simulink model "AppMain"  (R2021a)
settings: Solver=FixedStepDiscrete  StartTime=0.0  StopTime=80  FixedStep=10e-3  RelTol=1e-3
PreLoadFcn:
  | AppMain_data
values from neighbouring files (symbols this model uses):
  CtrlConst = struct    [AppMain_data.m]
  TaskTimeBase = struct    [AppMain_data.m]
undefined symbols (not defined in the file or in its folder): Lock, Open, Short
libraries: simulink x27, lib1 x10
(part 2 of 3)

== system AppMain/MotorRestartAndFaultCnt/MotorFalutHandle/Subsystem1 ==
  IsMotorShort : Inport  OutDataTypeStr=boolean
  IsMotorOpenLoad : Inport  Port=2  OutDataTypeStr=boolean
  TargetSpeed : Inport  Port=3  OutDataTypeStr=int16
  RestartEnable : Inport  Port=4  OutDataTypeStr=boolean
  If : If  IfExpression=u1 ~= 0
  If Action Subsystem : Subsystem  TreatAsAtomicUnit=on
  If Action Subsystem1 : Subsystem  TreatAsAtomicUnit=on
  Logical Operator : Logic  Operator=OR  AllPortsSameDT=off  OutDataTypeStr=boolean
  Merge : Merge
  Speed : Outport  OutDataTypeStr=int16  VectorParamsAs1DForOutWhenUnconnected=off
  wires:
  IsMotorShort/1 -> Logical Operator/1
  IsMotorOpenLoad/1 -> Logical Operator/2
  Logical Operator/1 -> If/1
  TargetSpeed/1 -> If Action Subsystem1/1(SpeedIn), If Action Subsystem/1(SpeedIn)
  RestartEnable/1 -> If Action Subsystem1/2(RestartEnable)
  If/1 -> If Action Subsystem/Action
  If/2 -> If Action Subsystem1/Action
  If Action Subsystem1/1(SpeedOut) -> Merge/2
  If Action Subsystem/1(SpeedOut) -> Merge/1
  Merge/1 -> Speed/1

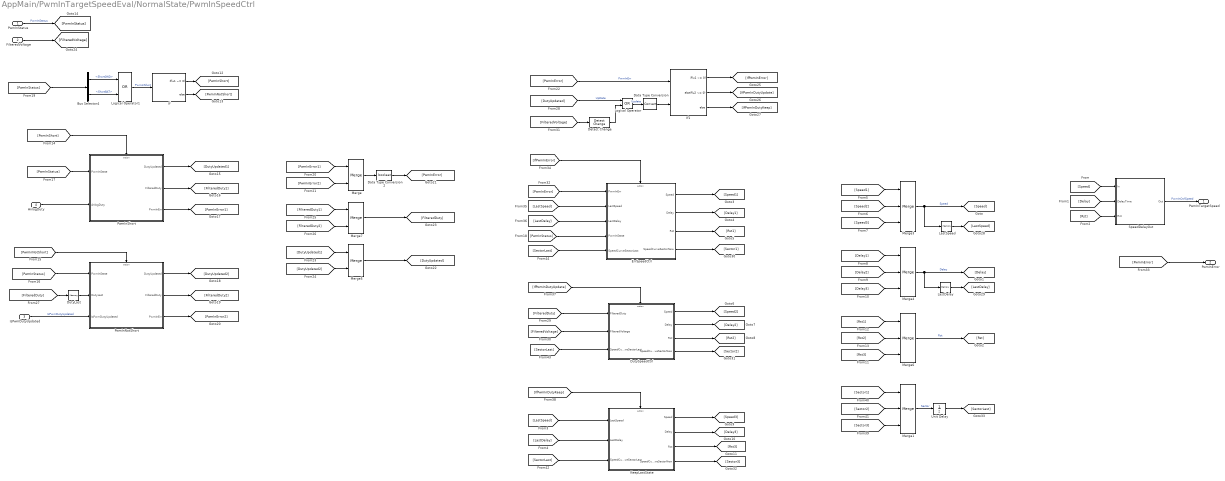
== system AppMain/PwmInTargetSpeedEval/NormalState/PwmInSpeedCtrl ==
  PwmInStatus : Inport
  FilteredVoltage : Inport  Port=2  OutDataTypeStr=int16
  IsPwmDutyUpdated : Inport  Port=3  OutDataTypeStr=boolean
  AnlogDuty : Inport  Port=4  OutDataTypeStr=uint16
  Bus Selector4 : BusSelector  OutputSignals=ShortGND,ShortBAT
  Data Type Conversion : DataTypeConversion
  Data Type Conversion2 : DataTypeConversion  OutDataTypeStr=boolean
  Detect Change : simulink/Logic and Bit Operations/Detect Change  vinit=0  OutDataTypeStr=boolean
  DutyLast : Memory  InitialCondition=CtrlConst.SpeedCtrl.PwmIn.Duty.Default  InheritSampleTime=on
  DutySpeedCtrl : Subsystem  TreatAsAtomicUnit=on
  ErrSpeedCtrl : Subsystem  TreatAsAtomicUnit=on
  If : If  IfExpression=u1 ~= 0
  If1 : If  NumInputs=2  IfExpression=u1 ~= 0  ElseIfExpressions=u2 ~= 0
  KeepLastState : Subsystem  TreatAsAtomicUnit=on
  LastDelay : Memory  InheritSampleTime=on
  LastSpeed : Memory  InheritSampleTime=on
  Logical Operator : Logic  Operator=OR  AllPortsSameDT=off  OutDataTypeStr=boolean
  Logical Operator1 : Logic  Operator=OR  AllPortsSameDT=off  OutDataTypeStr=boolean
  Merge : Merge
  Merge{1,3..4,6} (4 alike) : Merge  Inputs=3
  Merge5 : Merge
  Merge7 : Merge
  PwmInNotShort : Subsystem  TreatAsAtomicUnit=on
      settings: RTWSystemCode=Nonreusable function  RTWFcnNameOpts=Use subsystem name  FunctionInterfaceSpec=Allow arguments (Optimized)
  PwmInShort : Subsystem  TreatAsAtomicUnit=on
      settings: RTWSystemCode=Nonreusable function  RTWFcnNameOpts=Use subsystem name  FunctionInterfaceSpec=Allow arguments (Optimized)
  SpeedDelayOut : Subsystem  TreatAsAtomicUnit=on
      settings: RTWFcnNameOpts=Use subsystem name
  Unit Delay : UnitDelay  InitialCondition=CtrlConst.SpeedCtrl.DefaultSector  SampleTime=-1  HasFrameUpgradeWarning=on
  PwmInTargetSpeed : Outport  VectorParamsAs1DForOutWhenUnconnected=off
  PwmInError : Outport  Port=2  OutDataTypeStr=boolean  VectorParamsAs1DForOutWhenUnconnected=off
  wires:
  SpeedDelayOut/1(Out) -> PwmInTargetSpeed/1  "PwmInCtrlSpeed"
  PwmInStatus/1 -> [PwmInStatus]  "PwmInStatus"
  Bus Selector4/1 -> Logical Operator1/1  "<ShortGND>"
  Bus Selector4/2 -> Logical Operator1/2  "<ShortBAT>"
  Logical Operator1/1 -> If/1  "PwmInShort"
  [PwmInShort] -> PwmInShort/Action
  [PwmInNotShort] -> PwmInNotShort/Action
  [FilteredDuty] -> DutySpeedCtrl/1(FilteredDuty)
  Merge3/1 -> LastSpeed/1, [Speed]  "Speed"
  Merge4/1 -> LastDelay/1, [Delay]  "Delay"
  [DutyUpdated] -> Logical Operator/1  "UpDate"
  [LastDelay] -> KeepLastState/2(LastDelay)
  [LastSpeed] -> KeepLastState/1(LastSpeed)
  [PwmInError] -> If1/1  "PwmInErr"
  Data Type Conversion/1 -> If1/2
  DutyLast/1 -> PwmInNotShort/2(DutyLast)
  [FilteredVoltage] -> DutySpeedCtrl/2(FilteredVoltage)
  Merge/1 -> Data Type Conversion2/1
  Logical Operator/1 -> Data Type Conversion/1  "Update"
  IsPwmDutyUpdated/1 -> PwmInNotShort/3(IsPwmDutyUpdated)  "IsPwmDutyUpdated"
  AnlogDuty/1 -> PwmInShort/2(AnlogDuty)
  Merge6/1 -> [Rst]  "Rst"
  [Speed] -> SpeedDelayOut/1(In)
  [Delay] -> SpeedDelayOut/2(DelayTime)
  [Rst] -> SpeedDelayOut/3(Rst)
  ErrSpeedCtrl/1(Speed) -> [Speed1]
  ErrSpeedCtrl/2(Delay) -> [Delay1]
  ErrSpeedCtrl/3(Rst) -> [Rst1]
  DutySpeedCtrl/1(Speed) -> [Speed2]
  DutySpeedCtrl/2(Delay) -> [Delay2]
  DutySpeedCtrl/3(Rst) -> [Rst2]
  KeepLastState/1(Speed) -> [Speed3]
  KeepLastState/2(Delay) -> [Delay3]
  KeepLastState/3(Rst) -> [Rst3]
  [Speed1] -> Merge3/1
  [Speed2] -> Merge3/2
  [Speed3] -> Merge3/3
  [Delay1] -> Merge4/1
  [Delay2] -> Merge4/2
  [Delay3] -> Merge4/3
  [Rst3] -> Merge6/3
  [Rst2] -> Merge6/2
  [Rst1] -> Merge6/1
  If/1 -> [PwmInShort]
  If/2 -> [PwmInNotShort]
  [PwmInStatus] -> PwmInNotShort/1(PwmInState)
  [PwmInStatus] -> ErrSpeedCtrl/4(PwmInState)
  [PwmInStatus] -> PwmInShort/1(PwmInState)
  [PwmInStatus] -> Bus Selector4/1
  PwmInShort/3(PwmInErr) -> [PwmInError1]
  PwmInShort/2(FilteredDuty) -> [FilteredDuty1]
  PwmInShort/1(DutyUpdated) -> [DutyUpdated1]
  PwmInNotShort/1(DutyUpdated) -> [DutyUpdated2]
  PwmInNotShort/2(FilteredDuty) -> [FilteredDuty2]
  PwmInNotShort/3(PwmInErr) -> [PwmInError2]
  [PwmInError1] -> Merge/1
  [PwmInError2] -> Merge/2
  [DutyUpdated2] -> Merge5/2
  [DutyUpdated1] -> Merge5/1
  Merge5/1 -> [DutyUpdated]
  Merge7/1 -> [FilteredDuty]
  [FilteredDuty1] -> Merge7/1
  [FilteredDuty2] -> Merge7/2
  [FilteredDuty] -> DutyLast/1
  [FilteredVoltage] -> Detect Change/1
  Detect Change/1 -> Logical Operator/2
  FilteredVoltage/1 -> [FilteredVoltage]
  Data Type Conversion2/1 -> [PwmInError]
  [PwmInError] -> ErrSpeedCtrl/1(PwmInErr)
  [PwmInError] -> PwmInError/1
  If1/1 -> [IfPwmInError]
  If1/2 -> [IfPwmInDutyUpdate]
  If1/3 -> [IfPwmInDutyKeep]
  [IfPwmInError] -> ErrSpeedCtrl/Action
  LastSpeed/1 -> [LastSpeed]
  LastDelay/1 -> [LastDelay]
  [LastSpeed] -> ErrSpeedCtrl/2(LastSpeed)
  [LastDelay] -> ErrSpeedCtrl/3(LastDelay)
  ErrSpeedCtrl/4(SpeedCurveSectorNew) -> [Sector1]
  [IfPwmInDutyUpdate] -> DutySpeedCtrl/Action
  DutySpeedCtrl/4(SpeedCurveSectorNew) -> [Sector2]
  [IfPwmInDutyKeep] -> KeepLastState/Action
  KeepLastState/4(SpeedCurveSectorNew) -> [Sector3]
  [Sector1] -> Merge1/1
  [Sector2] -> Merge1/2
  [Sector3] -> Merge1/3
  Merge1/1 -> Unit Delay/1  "Sector"
  Unit Delay/1 -> [SectorLast]
  [SectorLast] -> KeepLastState/3(SpeedCurveSectorLast)
  [SectorLast] -> DutySpeedCtrl/3(SpeedCurveSectorLast)
  [SectorLast] -> ErrSpeedCtrl/5(SpeedCurveSectorLast)

== system AppMain/FeedBack/Subsystem7/Subsystem10/Subsystem1 ==
  Status : Inport
  Compare To Zero : simulink/Logic and Bit Operations/Compare To Zero  relop=~=  OutDataTypeStr=boolean
  Constant1 : Constant  Value=CtrlConst.FeedBack.EndDelay.Voltage  OutDataTypeStr=uint16
  Constant2 : Constant  Value=CtrlConst.FeedBack.StartDelay.Voltage  OutDataTypeStr=uint16
  Display : Display
  Display1 : Display
  FeedBackDelay4 : lib1/FeedBackDelay  SystemSampleTime=-1  VariantActivationTime=update diagram  Latency=0  AutoFrameSizeCalculation=off
      settings: SourceProductName=lib1
  FeedBackFlag : Outport  VectorParamsAs1DForOutWhenUnconnected=off
  wires:
  FeedBackDelay4/1 -> FeedBackFlag/1  "FeedBackFlag"
  Constant1/1 -> Display1/1, FeedBackDelay4/3
  Constant2/1 -> Display/1, FeedBackDelay4/1
  Compare To Zero/1 -> FeedBackDelay4/2
  Status/1 -> Compare To Zero/1

== system AppMain/FeedBack/Subsystem7/Subsystem10/Subsystem2 ==
  Status : Inport
  Compare To Zero : simulink/Logic and Bit Operations/Compare To Zero  relop=>  OutDataTypeStr=boolean
  Constant1 : Constant  Value=CtrlConst.FeedBack.EndDelay.AmbT  OutDataTypeStr=uint16
  Constant2 : Constant  Value=CtrlConst.FeedBack.StartDelay.AmbT  OutDataTypeStr=uint16
  Display : Display
  Display1 : Display
  FeedBackDelay4 : lib1/FeedBackDelay  SystemSampleTime=-1  VariantActivationTime=update diagram  Latency=0  AutoFrameSizeCalculation=off
      settings: SourceProductName=lib1
  FeedBackFlag : Outport  VectorParamsAs1DForOutWhenUnconnected=off
  wires:
  Status/1 -> Compare To Zero/1
  Compare To Zero/1 -> FeedBackDelay4/2
  Constant2/1 -> FeedBackDelay4/1, Display/1
  Constant1/1 -> FeedBackDelay4/3, Display1/1
  FeedBackDelay4/1 -> FeedBackFlag/1  "FeedBackFlag"

== system AppMain/FeedBack/Subsystem7/Subsystem10/Subsystem6 ==
  Status : Inport
  Compare To Zero : simulink/Logic and Bit Operations/Compare To Zero  relop=~=  OutDataTypeStr=boolean
  Constant1 : Constant  Value=CtrlConst.FeedBack.EndDelay.AmbTPreOver  OutDataTypeStr=uint16
  Constant2 : Constant  Value=CtrlConst.FeedBack.StartDelay.AmbTPreOver  OutDataTypeStr=uint16
  Display : Display
  Display1 : Display
  FeedBackDelay4 : lib1/FeedBackDelay  SystemSampleTime=-1  VariantActivationTime=update diagram  Latency=0  AutoFrameSizeCalculation=off
      settings: SourceProductName=lib1
  FeedBackFlag : Outport  VectorParamsAs1DForOutWhenUnconnected=off
  wires:
  Status/1 -> Compare To Zero/1
  Compare To Zero/1 -> FeedBackDelay4/2
  Constant2/1 -> FeedBackDelay4/1, Display/1
  Constant1/1 -> FeedBackDelay4/3, Display1/1
  FeedBackDelay4/1 -> FeedBackFlag/1  "FeedBackFlag"

== system AppMain/FeedBack/Subsystem7/Subsystem10/Subsystem7 ==
  Status : Inport
  Compare To Zero : simulink/Logic and Bit Operations/Compare To Zero  relop=~=  OutDataTypeStr=boolean
  Constant1 : Constant  Value=CtrlConst.FeedBack.EndDelay.MotorShort  OutDataTypeStr=uint16
  Constant2 : Constant  Value=CtrlConst.FeedBack.StartDelay.MotorShort  OutDataTypeStr=uint16
  Display : Display
  Display1 : Display
  FeedBackDelay4 : lib1/FeedBackDelay  SystemSampleTime=-1  VariantActivationTime=update diagram  Latency=0  AutoFrameSizeCalculation=off
      settings: SourceProductName=lib1
  FeedBackFlag : Outport  VectorParamsAs1DForOutWhenUnconnected=off
  wires:
  FeedBackDelay4/1 -> FeedBackFlag/1  "FeedBackFlag"
  Constant1/1 -> Display1/1, FeedBackDelay4/3
  Constant2/1 -> Display/1, FeedBackDelay4/1
  Compare To Zero/1 -> FeedBackDelay4/2
  Status/1 -> Compare To Zero/1

== system AppMain/FeedBack/Subsystem7/Subsystem10/Subsystem8 ==
  Status : Inport
  Compare To Zero : simulink/Logic and Bit Operations/Compare To Zero  relop=~=  OutDataTypeStr=boolean
  Constant1 : Constant  Value=CtrlConst.FeedBack.EndDelay.MotorOpenLoad  OutDataTypeStr=uint16
  Constant2 : Constant  Value=CtrlConst.FeedBack.StartDelay.MotorOpenLoad  OutDataTypeStr=uint16
  Display : Display
  Display1 : Display
  FeedBackDelay4 : lib1/FeedBackDelay  SystemSampleTime=-1  VariantActivationTime=update diagram  Latency=0  AutoFrameSizeCalculation=off
      settings: SourceProductName=lib1
  FeedBackFlag : Outport  VectorParamsAs1DForOutWhenUnconnected=off
  wires:
  Status/1 -> Compare To Zero/1
  Compare To Zero/1 -> FeedBackDelay4/2
  Constant2/1 -> FeedBackDelay4/1, Display/1
  Constant1/1 -> FeedBackDelay4/3, Display1/1
  FeedBackDelay4/1 -> FeedBackFlag/1  "FeedBackFlag"

== system AppMain/FeedBack/Subsystem7/Subsystem10/Subsystem9 ==
  Status : Inport
  Compare To Zero : simulink/Logic and Bit Operations/Compare To Zero  relop=~=  OutDataTypeStr=boolean
  Constant1 : Constant  Value=CtrlConst.FeedBack.EndDelay.MotorLock  OutDataTypeStr=uint16
  Constant2 : Constant  Value=CtrlConst.FeedBack.StartDelay.MotorLock  OutDataTypeStr=uint16
  Display : Display
  Display1 : Display
  FeedBackDelay4 : lib1/FeedBackDelay  SystemSampleTime=-1  VariantActivationTime=update diagram  Latency=0  AutoFrameSizeCalculation=off
      settings: SourceProductName=lib1
  FeedBackFlag : Outport  VectorParamsAs1DForOutWhenUnconnected=off
  wires:
  FeedBackDelay4/1 -> FeedBackFlag/1  "FeedBackFlag"
  Constant1/1 -> Display1/1, FeedBackDelay4/3
  Constant2/1 -> Display/1, FeedBackDelay4/1
  Compare To Zero/1 -> FeedBackDelay4/2
  Status/1 -> Compare To Zero/1

== system AppMain/MotorRestartAndFaultCnt/MotorFalutHandle/Subsystem/If Action Subsystem ==
  FalutCntLast : Inport  OutDataTypeStr=Bus: MotorFaultCnt_t
  IsMotorShort : Inport  Port=2  OutDataTypeStr=boolean
  IsMotorLock : Inport  Port=3  OutDataTypeStr=boolean
  IsMotorOpenLoad : Inport  Port=4  OutDataTypeStr=boolean
  Action Port : ActionPort  InitializeStates=reset  ActionPortLabel=if(u1 ~= 0)
  FaultCntIncrement : Subsystem
  RestartIntervalCaculate : Subsystem
  FaultCnt : Outport  OutDataTypeStr=Bus: MotorFaultCnt_t  VectorParamsAs1DForOutWhenUnconnected=off
  RestartInterval : Outport  Port=2  OutDataTypeStr=uint16  VectorParamsAs1DForOutWhenUnconnected=off
  wires:
  FaultCntIncrement/1(FaultCnt) -> RestartIntervalCaculate/1(MotorFaultCnt), FaultCnt/1
  FalutCntLast/1 -> FaultCntIncrement/1(FalutCntLast)
  IsMotorShort/1 -> FaultCntIncrement/2(IsMotorShort)
  RestartIntervalCaculate/1(TimeTHR) -> RestartInterval/1
  IsMotorOpenLoad/1 -> FaultCntIncrement/3(IsMotorOpenLoad)
  IsMotorLock/1 -> FaultCntIncrement/4(IsMotorLock)

== system AppMain/MotorRestartAndFaultCnt/MotorFalutHandle/Subsystem/If Action Subsystem1 ==
  FaultCntLast : Inport  OutDataTypeStr=Bus: MotorFaultCnt_t
  RestartIntervalLast : Inport  Port=2  OutDataTypeStr=uint16
  Action Port : ActionPort  InitializeStates=reset  ActionPortLabel=else
  Bus Creator : BusCreator  Inputs=3  OutDataTypeStr=Bus: MotorFaultCnt_t  NonVirtualBus=on
      settings: InheritFromInputs=off
  Bus Selector : BusSelector  OutputSignals=Short,Open,Lock
  FaultCnt : Outport  OutDataTypeStr=Bus: MotorFaultCnt_t  VectorParamsAs1DForOutWhenUnconnected=off
  RestartInterval : Outport  Port=2  OutDataTypeStr=uint16  VectorParamsAs1DForOutWhenUnconnected=off
  wires:
  FaultCntLast/1 -> Bus Selector/1
  Bus Creator/1 -> FaultCnt/1
  Bus Selector/1 -> Bus Creator/1  "<Short>"
  Bus Selector/2 -> Bus Creator/2  "<Open>"
  Bus Selector/3 -> Bus Creator/3  "<Lock>"
  RestartIntervalLast/1 -> RestartInterval/1

== system AppMain/MotorRestartAndFaultCnt/MotorFalutHandle/Subsystem1/If Action Subsystem ==
  SpeedIn : Inport
  Action Port : ActionPort  ActionPortLabel=if(u1 ~= 0)
  SpeedOut : Outport  VectorParamsAs1DForOutWhenUnconnected=off
  wires:
  SpeedIn/1 -> SpeedOut/1

== system AppMain/MotorRestartAndFaultCnt/MotorFalutHandle/Subsystem1/If Action Subsystem1 ==
  SpeedIn : Inport
  RestartEnable : Inport  Port=2  OutDataTypeStr=boolean
  Action Port : ActionPort  InitializeStates=reset  ActionPortLabel=else
  Terminator : Terminator
  SpeedOut : Outport  VectorParamsAs1DForOutWhenUnconnected=off
  wires:
  SpeedIn/1 -> SpeedOut/1
  RestartEnable/1 -> Terminator/1

== system AppMain/PwmInTargetSpeedEval/NormalState/PwmInSpeedCtrl/DutySpeedCtrl ==
  FilteredDuty : Inport  OutDataTypeStr=uint16
  FilteredVoltage : Inport  Port=2  OutDataTypeStr=int16
  SpeedCurveSectorLast : Inport  Port=3
  Action Port : ActionPort  InitializeStates=reset  ActionPortLabel=elseif(u2 ~= 0)
  SpeedAndOutDelayEval : Subsystem
      settings: RTWFcnNameOpts=Use subsystem name
  Speed : Outport  OutDataTypeStr=int16  VectorParamsAs1DForOutWhenUnconnected=off
  Delay : Outport  Port=2  OutDataTypeStr=uint16  VectorParamsAs1DForOutWhenUnconnected=off
  Rst : Outport  Port=3  OutDataTypeStr=boolean  VectorParamsAs1DForOutWhenUnconnected=off
  SpeedCurveSectorNew : Outport  Port=4
  wires:
  FilteredDuty/1 -> SpeedAndOutDelayEval/1(FilteredDuty)
  SpeedAndOutDelayEval/1(DutySpeed) -> Speed/1  "Speed"
  SpeedAndOutDelayEval/2(DelayTime) -> Delay/1  "Delay"
  SpeedAndOutDelayEval/3(DelayRst) -> Rst/1  "Rst"
  FilteredVoltage/1 -> SpeedAndOutDelayEval/2(FilteredVoltage)
  SpeedCurveSectorLast/1 -> SpeedAndOutDelayEval/3(SpeedCurveSectorLast)
  SpeedAndOutDelayEval/4(SpeedCurveSectorNew) -> SpeedCurveSectorNew/1

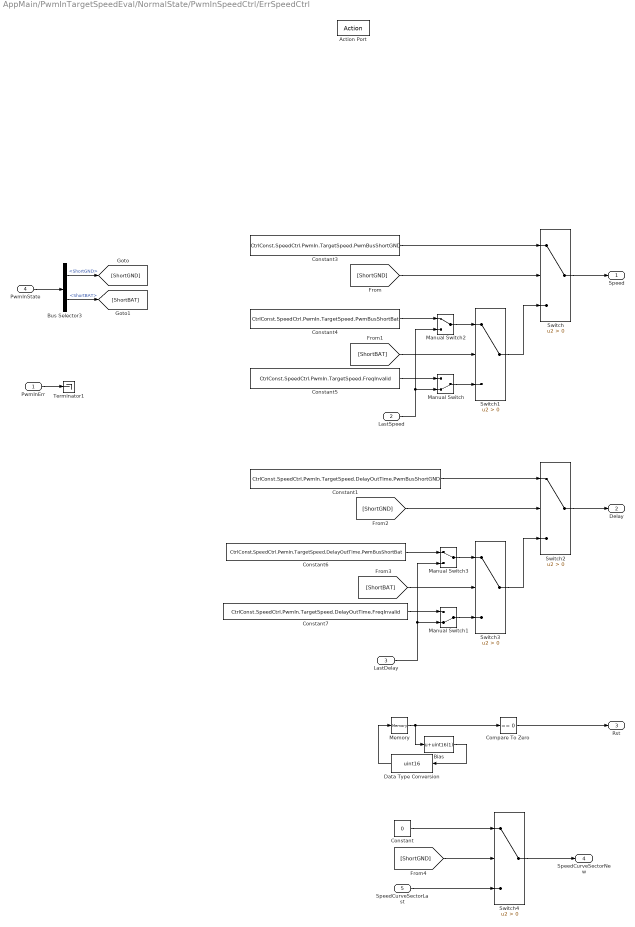
== system AppMain/PwmInTargetSpeedEval/NormalState/PwmInSpeedCtrl/ErrSpeedCtrl ==
  PwmInErr : Inport  OutDataTypeStr=boolean
  LastSpeed : Inport  Port=2  OutDataTypeStr=int16
  LastDelay : Inport  Port=3  OutDataTypeStr=uint16
  PwmInState : Inport  Port=4
  SpeedCurveSectorLast : Inport  Port=5
  Action Port : ActionPort  InitializeStates=reset  ActionPortLabel=if(u1 ~= 0)
  Bias : Bias  Bias=uint16(1)
  Bus Selector3 : BusSelector  OutputSignals=ShortGND,ShortBAT
  Compare To Zero : simulink/Logic and Bit Operations/Compare To Zero  relop===  OutDataTypeStr=boolean
  Constant : Constant  Value=0  OutDataTypeStr=uint16
  Constant1 : Constant  Value=CtrlConst.SpeedCtrl.PwmIn.TargetSpeed.DelayOutTime.PwmBusShortGND
  Constant3 : Constant  Value=CtrlConst.SpeedCtrl.PwmIn.TargetSpeed.PwmBusShortGND
  Constant4 : Constant  Value=CtrlConst.SpeedCtrl.PwmIn.TargetSpeed.PwmBusShortBat
  Constant5 : Constant  Value=CtrlConst.SpeedCtrl.PwmIn.TargetSpeed.FreqInvalid
  Constant6 : Constant  Value=CtrlConst.SpeedCtrl.PwmIn.TargetSpeed.DelayOutTime.PwmBusShortBat
  Constant7 : Constant  Value=CtrlConst.SpeedCtrl.PwmIn.TargetSpeed.DelayOutTime.FreqInvalid
  Data Type Conversion : DataTypeConversion  OutDataTypeStr=uint16
  Manual Switch : ManualSwitch  CurrentSetting=0
  Manual Switch1 : ManualSwitch  CurrentSetting=0
  Manual Switch2 : ManualSwitch
  Manual Switch3 : ManualSwitch
  Memory : Memory  InitialCondition=uint16(0)  InheritSampleTime=on
  Switch{,1..4} (5 alike) : Switch  Criteria=u2 > Threshold
  Terminator1 : Terminator
  Speed : Outport  OutDataTypeStr=int16  VectorParamsAs1DForOutWhenUnconnected=off
  Delay : Outport  Port=2  OutDataTypeStr=uint16  VectorParamsAs1DForOutWhenUnconnected=off
  Rst : Outport  Port=3  OutDataTypeStr=boolean  VectorParamsAs1DForOutWhenUnconnected=off
  SpeedCurveSectorNew : Outport  Port=4  OutDataTypeStr=uint16
  wires:
  PwmInState/1 -> Bus Selector3/1
  Constant3/1 -> Switch/1
  Switch1/1 -> Switch/3
  Switch/1 -> Speed/1
  Switch3/1 -> Switch2/3
  Constant1/1 -> Switch2/1
  Switch2/1 -> Delay/1
  Data Type Conversion/1 -> Memory/1
  Bias/1 -> Data Type Conversion/1
  Memory/1 -> Bias/1, Compare To Zero/1
  Compare To Zero/1 -> Rst/1
  LastSpeed/1 -> Manual Switch2/2, Manual Switch/2
  LastDelay/1 -> Manual Switch3/2, Manual Switch1/2
  Constant4/1 -> Manual Switch2/1
  PwmInErr/1 -> Terminator1/1
  Manual Switch/1 -> Switch1/3
  Constant5/1 -> Manual Switch/1
  Constant7/1 -> Manual Switch1/1
  Manual Switch1/1 -> Switch3/3
  Manual Switch2/1 -> Switch1/1
  Constant6/1 -> Manual Switch3/1
  Switch4/1 -> SpeedCurveSectorNew/1
  Bus Selector3/1 -> [ShortGND]  "<ShortGND>"
  Bus Selector3/2 -> [ShortBAT]  "<ShortBAT>"
  [ShortGND] -> Switch/2
  [ShortBAT] -> Switch1/2
  [ShortGND] -> Switch2/2
  [ShortBAT] -> Switch3/2
  [ShortGND] -> Switch4/2
  Constant/1 -> Switch4/1
  SpeedCurveSectorLast/1 -> Switch4/3
  Manual Switch3/1 -> Switch3/1

== system AppMain/PwmInTargetSpeedEval/NormalState/PwmInSpeedCtrl/KeepLastState ==
  LastSpeed : Inport  OutDataTypeStr=int16
  LastDelay : Inport  Port=2  OutDataTypeStr=uint16
  SpeedCurveSectorLast : Inport  Port=3  OutDataTypeStr=uint16
  Action Port : ActionPort  InitializeStates=reset  ActionPortLabel=else
  Constant : Constant  Value=false  OutDataTypeStr=boolean
  Speed : Outport  OutDataTypeStr=int16  VectorParamsAs1DForOutWhenUnconnected=off
  Delay : Outport  Port=2  OutDataTypeStr=uint16  VectorParamsAs1DForOutWhenUnconnected=off
  Rst : Outport  Port=3  OutDataTypeStr=boolean  VectorParamsAs1DForOutWhenUnconnected=off
  SpeedCurveSectorNew : Outport  Port=4  OutDataTypeStr=uint16
  wires:
  LastSpeed/1 -> Speed/1
  LastDelay/1 -> Delay/1
  Constant/1 -> Rst/1
  SpeedCurveSectorLast/1 -> SpeedCurveSectorNew/1

== system AppMain/PwmInTargetSpeedEval/NormalState/PwmInSpeedCtrl/PwmInNotShort ==
  PwmInState : Inport
  DutyLast : Inport  Port=2  OutDataTypeStr=uint16
  IsPwmDutyUpdated : Inport  Port=3  OutDataTypeStr=boolean
  Action Port : ActionPort  InitializeStates=reset  ActionPortLabel=else
  Bus Selector2 : BusSelector  OutputSignals=Freq,HighDuty
  Detect Increase : simulink/Logic and Bit Operations/Detect Increase  vinit=0.0  OutDataTypeStr=boolean
  DutyFilter : Subsystem  TreatAsAtomicUnit=on
      settings: RTWFcnNameOpts=Use subsystem name
  FreqValidJudge : Subsystem  TreatAsAtomicUnit=on
      settings: RTWFcnNameOpts=Use subsystem name
  Logical Operator : Logic  Operator=OR  AllPortsSameDT=off  OutDataTypeStr=boolean
  Logical Operator2 : Logic  Operator=NOT  Inputs=3  AllPortsSameDT=off  OutDataTypeStr=boolean
  Relational Operator : RelationalOperator  Operator=~=  OutDataTypeStr=boolean  RndMeth=Simplest
  Switch : Switch  Criteria=u2 > Threshold
  DutyUpdated : Outport  OutDataTypeStr=boolean  VectorParamsAs1DForOutWhenUnconnected=off
  FilteredDuty : Outport  Port=2  OutDataTypeStr=uint16  VectorParamsAs1DForOutWhenUnconnected=off
  PwmInErr : Outport  Port=3  OutDataTypeStr=boolean  VectorParamsAs1DForOutWhenUnconnected=off
  wires:
  Detect Increase/1 -> Logical Operator/1
  DutyFilter/2(Valid) -> Detect Increase/1  "Valid"
  PwmInState/1 -> Bus Selector2/1
  Bus Selector2/2 -> DutyFilter/1(Duty)  "<HighDuty>"
  Bus Selector2/1 -> FreqValidJudge/1(Freq)  "<Freq>"
  DutyFilter/1(FilteredDuty) -> Relational Operator/1, Switch/1  "FilteredDuty"
  Logical Operator2/1 -> PwmInErr/1  "FreqInvalid"
  FreqValidJudge/1(Valid) -> Logical Operator2/1, Switch/2, DutyFilter/Enable  "FreqValid"
  Relational Operator/1 -> Logical Operator/2
  Logical Operator/1 -> DutyUpdated/1  "UpdateFlag"
  IsPwmDutyUpdated/1 -> DutyFilter/3(IsPwmDutyUpdated)  "IsPwmDutyUpdated"
  Switch/1 -> FilteredDuty/1
  DutyLast/1 -> Relational Operator/2, Switch/3, DutyFilter/2(DutyLast)  "FilteredDuty"

== system AppMain/PwmInTargetSpeedEval/NormalState/PwmInSpeedCtrl/PwmInShort ==
  PwmInState : Inport
  AnlogDuty : Inport  Port=2  OutDataTypeStr=uint16
  Action Port : ActionPort  InitializeStates=reset  ActionPortLabel=if(u1 ~= 0)
  Bus Selector3 : BusSelector  OutputSignals=ShortGND,ShortBAT
  Constant : Constant  Value=true  OutDataTypeStr=boolean
  Detect Change : simulink/Logic and Bit Operations/Detect Change  vinit=0  OutDataTypeStr=boolean
  Detect Increase : simulink/Logic and Bit Operations/Detect Increase  vinit=0.0  OutDataTypeStr=boolean
  Detect Increase1 : simulink/Logic and Bit Operations/Detect Increase  vinit=0.0  OutDataTypeStr=boolean
  Duty0 : Constant  Value=0  OutDataTypeStr=uint16
  Duty100 : Constant  Value=1000  OutDataTypeStr=uint16
  Logical Operator3 : Logic  Operator=OR  Inputs=3  AllPortsSameDT=off  OutDataTypeStr=boolean
  Manual Switch : ManualSwitch  CurrentSetting=0
  Switch : Switch  Criteria=u2 > Threshold
  DutyUpdated : Outport  OutDataTypeStr=boolean  VectorParamsAs1DForOutWhenUnconnected=off
  FilteredDuty : Outport  Port=2  OutDataTypeStr=uint16  VectorParamsAs1DForOutWhenUnconnected=off
  PwmInErr : Outport  Port=3  OutDataTypeStr=boolean  VectorParamsAs1DForOutWhenUnconnected=off
  wires:
  Switch/1 -> FilteredDuty/1  "FilteredDuty"
  Logical Operator3/1 -> DutyUpdated/1  "DutyUpdate"
  Bus Selector3/2 -> Detect Increase1/1, Switch/2  "<ShortBAT>"
  Bus Selector3/1 -> Detect Increase/1  "<ShortGND>"
  Detect Increase1/1 -> Logical Operator3/2
  Detect Increase/1 -> Logical Operator3/1
  Duty0/1 -> Switch/1
  PwmInState/1 -> Bus Selector3/1
  Constant/1 -> PwmInErr/1
  AnlogDuty/1 -> Manual Switch/1, Detect Change/1
  Detect Change/1 -> Logical Operator3/3
  Manual Switch/1 -> Switch/3
  Duty100/1 -> Manual Switch/2

== system AppMain/PwmInTargetSpeedEval/NormalState/PwmInSpeedCtrl/SpeedDelayOut ==
  In : Inport
  DelayTime : Inport  Port=2
  Rst : Inport  Port=3
  DelayOut : Stateflow chart  TreatAsAtomicUnit=on
  OutLast : Memory  InheritSampleTime=on
  Out : Outport  VectorParamsAs1DForOutWhenUnconnected=off
  wires:
  In/1 -> DelayOut/1(In)  "In"
  OutLast/1 -> DelayOut/4(OutLast)  "OutLast"
  Rst/1 -> DelayOut/3(Rst)  "Rst"
  DelayOut/1(Out) -> OutLast/1, Out/1  "Out"
  DelayTime/1 -> DelayOut/2(DelayTHR)  "DelayTHR"

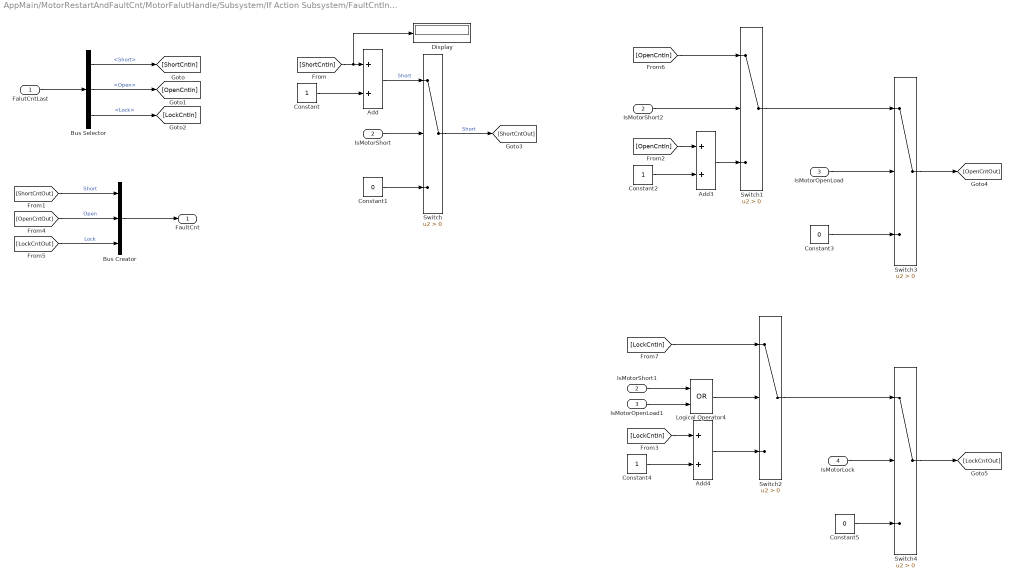
== system AppMain/MotorRestartAndFaultCnt/MotorFalutHandle/Subsystem/If Action Subsystem/FaultCntIncrement ==
  FalutCntLast : Inport  OutDataTypeStr=Bus: MotorFaultCnt_t
  IsMotorShort : Inport  Port=2  OutDataTypeStr=boolean
  IsMotorOpenLoad : Inport  Port=3  OutDataTypeStr=boolean
  IsMotorLock : Inport  Port=4  OutDataTypeStr=boolean
  Add : Sum  SaturateOnIntegerOverflow=on
  Add3 : Sum  SaturateOnIntegerOverflow=on
  Add4 : Sum  SaturateOnIntegerOverflow=on
  Bus Creator : BusCreator  Inputs=Short,Open,Lock  OutDataTypeStr=Bus: MotorFaultCnt_t  NonVirtualBus=on
  Bus Selector : BusSelector  OutputSignals=Short,Open,Lock
  Constant : Constant  OutDataTypeStr=uint8
  Constant1 : Constant  Value=0  OutDataTypeStr=uint8
  Constant2 : Constant  OutDataTypeStr=uint8
  Constant3 : Constant  Value=0  OutDataTypeStr=uint8
  Constant4 : Constant  OutDataTypeStr=uint8
  Constant5 : Constant  Value=0  OutDataTypeStr=uint8
  Display : Display
  IsMotorOpenLoad1 : InportShadow  Port=3  OutDataTypeStr=boolean
  IsMotorShort1 : InportShadow  Port=2  OutDataTypeStr=boolean
  IsMotorShort2 : InportShadow  Port=2  OutDataTypeStr=boolean
  Logical Operator4 : Logic  Operator=OR  AllPortsSameDT=off  OutDataTypeStr=boolean
  Switch{,1..4} (5 alike) : Switch  Criteria=u2 > Threshold
  FaultCnt : Outport  OutDataTypeStr=Bus: MotorFaultCnt_t  VectorParamsAs1DForOutWhenUnconnected=off
  wires:
  Bus Creator/1 -> FaultCnt/1
  Constant/1 -> Add/2
  Bus Selector/2 -> [OpenCntIn]  "<Open>"
  Bus Selector/1 -> [ShortCntIn]  "<Short>"
  Constant1/1 -> Switch/3
  Add/1 -> Switch/1  "Short"
  FalutCntLast/1 -> Bus Selector/1
  IsMotorShort/1 -> Switch/2
  Bus Selector/3 -> [LockCntIn]  "<Lock>"
  [ShortCntIn] -> Display/1, Add/1
  Switch/1 -> [ShortCntOut]  "Short"
  [ShortCntOut] -> Bus Creator/1  "Short"
  Add3/1 -> Switch1/3
  Constant2/1 -> Add3/2
  [OpenCntIn] -> Add3/1
  Constant3/1 -> Switch3/3
  Switch3/1 -> [OpenCntOut]
  IsMotorShort1/1 -> Logical Operator4/1
  Switch4/1 -> [LockCntOut]
  [LockCntIn] -> Add4/1
  Constant4/1 -> Add4/2
  Constant5/1 -> Switch4/3
  IsMotorOpenLoad1/1 -> Logical Operator4/2
  [OpenCntOut] -> Bus Creator/2  "Open"
  [LockCntOut] -> Bus Creator/3  "Lock"
  IsMotorOpenLoad/1 -> Switch3/2
  IsMotorShort2/1 -> Switch1/2
  [OpenCntIn] -> Switch1/1
  Switch1/1 -> Switch3/1
  IsMotorLock/1 -> Switch4/2
  Switch2/1 -> Switch4/1
  Logical Operator4/1 -> Switch2/2
  [LockCntIn] -> Switch2/1
  Add4/1 -> Switch2/3

== system AppMain/MotorRestartAndFaultCnt/MotorFalutHandle/Subsystem/If Action Subsystem/RestartIntervalCaculate ==
  MotorFaultCnt : Inport  OutDataTypeStr=Bus: MotorFaultCnt_t
  Bus Selector : BusSelector  OutputSignals=Short,Open,Lock
  If : If  NumInputs=2  ElseIfExpressions=u2 > 0
  Lock : Subsystem  TreatAsAtomicUnit=on
  Merge : Merge  Inputs=3
  Open : Subsystem  TreatAsAtomicUnit=on
  Scope : Scope  NumInputPorts=4
  Short : Subsystem  TreatAsAtomicUnit=on
  TimeTHR : Outport  OutDataTypeStr=uint16  VectorParamsAs1DForOutWhenUnconnected=off
  wires:
  Bus Selector/1 -> If/1, Scope/2, Short/1(FaultCnt)  "<Short>"
  Bus Selector/3 -> Lock/1(FaultCnt), Scope/4  "<Lock>"
  Bus Selector/2 -> Open/1(FaultCnt), Scope/3, If/2  "<Open>"
  MotorFaultCnt/1 -> Bus Selector/1
  If/1 -> Short/Action
  If/2 -> Open/Action
  If/3 -> Lock/Action
  Merge/1 -> TimeTHR/1, Scope/1
  Open/1(Interval) -> Merge/2
  Lock/1(Interval) -> Merge/3
  Short/1(Interval) -> Merge/1

== system AppMain/PwmInTargetSpeedEval/NormalState/PwmInSpeedCtrl/DutySpeedCtrl/SpeedAndOutDelayEval ==
  FilteredDuty : Inport
  FilteredVoltage : Inport  Port=2  OutDataTypeStr=int16
  SpeedCurveSectorLast : Inport  Port=3
  Data Type Conversion : DataTypeConversion  OutDataTypeStr=int16
  MaxSpeedLimtedByVoltage : Subsystem  TreatAsAtomicUnit=on
  SpeedCurve : Subsystem  TreatAsAtomicUnit=on
  DutySpeed : Outport  VectorParamsAs1DForOutWhenUnconnected=off
  DelayTime : Outport  Port=2  VectorParamsAs1DForOutWhenUnconnected=off
  DelayRst : Outport  Port=3  OutDataTypeStr=boolean  VectorParamsAs1DForOutWhenUnconnected=off
  SpeedCurveSectorNew : Outport  Port=4
  wires:
  FilteredVoltage/1 -> MaxSpeedLimtedByVoltage/1(Voltage)
  FilteredDuty/1 -> SpeedCurve/2(Duty)  "FilteredDuty"
  SpeedCurveSectorLast/1 -> SpeedCurve/3(SectorIn)
  SpeedCurve/4(SectorOut) -> SpeedCurveSectorNew/1
  SpeedCurve/3(Rst) -> DelayRst/1
  SpeedCurve/2(DelayTime) -> DelayTime/1
  SpeedCurve/1(Speed) -> DutySpeed/1
  MaxSpeedLimtedByVoltage/1(MaxSpeed) -> Data Type Conversion/1
  Data Type Conversion/1 -> SpeedCurve/1(MaxSpeed)

== system AppMain/PwmInTargetSpeedEval/NormalState/PwmInSpeedCtrl/PwmInNotShort/DutyFilter ==
  Duty : Inport
  DutyLast : Inport  Port=2  OutDataTypeStr=uint16
  IsPwmDutyUpdated : Inport  Port=3  OutDataTypeStr=boolean
  Enable : EnablePort  StatesWhenEnabling=reset
  DutyBuf : Memory  InitialCondition=uint16(ones(1,6)*2000)  InheritSampleTime=on
  Enabled Subsystem : Subsystem  TreatAsAtomicUnit=on
  Switch : Switch  Criteria=u2 > Threshold
  FilteredDuty : Outport  VectorParamsAs1DForOutWhenUnconnected=off
  Valid : Outport  Port=2  VectorParamsAs1DForOutWhenUnconnected=off
  wires:
  Enabled Subsystem/2(Valid) -> Valid/1
  Duty/1 -> Enabled Subsystem/1(Duty)  "Duty"
  DutyLast/1 -> Switch/3, Enabled Subsystem/2(DutyLast)  "DutyLast"
  Enabled Subsystem/1(FilteredDuty) -> Switch/1
  IsPwmDutyUpdated/1 -> Enabled Subsystem/Enable, Switch/2  "IsPwmDutyUpdated"
  Enabled Subsystem/3(DutyBufOut) -> DutyBuf/1
  DutyBuf/1 -> Enabled Subsystem/3(DutyBufIn)
  Switch/1 -> FilteredDuty/1

== system AppMain/PwmInTargetSpeedEval/NormalState/PwmInSpeedCtrl/PwmInNotShort/FreqValidJudge ==
  Freq : Inport
  FreqMax : Constant  Value=CtrlConst.SpeedCtrl.PwmIn.Freq.Max
  FreqMin : Constant  Value=CtrlConst.SpeedCtrl.PwmIn.Freq.Min
  FreqTolerance : Constant  Value=CtrlConst.SpeedCtrl.PwmIn.Freq.Tolerance
  FreqValidJudge : Stateflow chart  TreatAsAtomicUnit=on
  FreqValidJudgeFilterTime : Constant  Value=CtrlConst.SpeedCtrl.PwmIn.Freq.ValidJudgeFilterTime
  Valid : Outport  VectorParamsAs1DForOutWhenUnconnected=off
  wires:
  FreqValidJudge/1(Valid) -> Valid/1
  Freq/1 -> FreqValidJudge/1(Freq)
  FreqMin/1 -> FreqValidJudge/2(FreqMin)
  FreqMax/1 -> FreqValidJudge/3(FreqMax)
  FreqTolerance/1 -> FreqValidJudge/4(FreqTolerance)
  FreqValidJudgeFilterTime/1 -> FreqValidJudge/5(FreqValidJudgeFilterTime)

== system AppMain/MotorRestartAndFaultCnt/MotorFalutHandle/Subsystem/If Action Subsystem/RestartIntervalCaculate/Lock ==
  FaultCnt : Inport
  Action Port : ActionPort  InitializeStates=reset  ActionPortLabel=else
  Constant3 : Constant  Value=5/TaskTimeBase.SpeedCtrl  OutDataTypeStr=uint16
  Constant4 : Constant  Value=18/TaskTimeBase.SpeedCtrl  OutDataTypeStr=uint16
  Constant5 : Constant  Value=33/TaskTimeBase.SpeedCtrl  OutDataTypeStr=uint16
  Constant6 : Constant  Value=60/TaskTimeBase.SpeedCtrl  OutDataTypeStr=uint16
  Multiport Switch : MultiPortSwitch  Inputs=4  DiagnosticForDefault=None
  Interval : Outport  VectorParamsAs1DForOutWhenUnconnected=off
  wires:
  Constant6/1 -> Multiport Switch/5
  Constant5/1 -> Multiport Switch/4
  FaultCnt/1 -> Multiport Switch/1
  Constant4/1 -> Multiport Switch/3
  Constant3/1 -> Multiport Switch/2
  Multiport Switch/1 -> Interval/1

== system AppMain/MotorRestartAndFaultCnt/MotorFalutHandle/Subsystem/If Action Subsystem/RestartIntervalCaculate/Open ==
  FaultCnt : Inport
  Action Port : ActionPort  InitializeStates=reset  ActionPortLabel=elseif(u2 > 0)
  Constant3 : Constant  Value=5/TaskTimeBase.SpeedCtrl  OutDataTypeStr=uint16
  Constant4 : Constant  Value=18/TaskTimeBase.SpeedCtrl  OutDataTypeStr=uint16
  Constant5 : Constant  Value=33/TaskTimeBase.SpeedCtrl  OutDataTypeStr=uint16
  Constant6 : Constant  Value=60/TaskTimeBase.SpeedCtrl  OutDataTypeStr=uint16
  Multiport Switch : MultiPortSwitch  Inputs=4  DiagnosticForDefault=None
  Interval : Outport  VectorParamsAs1DForOutWhenUnconnected=off
  wires:
  Constant6/1 -> Multiport Switch/5
  Constant5/1 -> Multiport Switch/4
  FaultCnt/1 -> Multiport Switch/1
  Constant4/1 -> Multiport Switch/3
  Constant3/1 -> Multiport Switch/2
  Multiport Switch/1 -> Interval/1

== system AppMain/MotorRestartAndFaultCnt/MotorFalutHandle/Subsystem/If Action Subsystem/RestartIntervalCaculate/Short ==
  FaultCnt : Inport
  Action Port : ActionPort  InitializeStates=reset  ActionPortLabel=if(u1 > 0)
  Constant3 : Constant  Value=5/TaskTimeBase.SpeedCtrl  OutDataTypeStr=uint16
  Constant4 : Constant  Value=18/TaskTimeBase.SpeedCtrl  OutDataTypeStr=uint16
  Constant5 : Constant  Value=33/TaskTimeBase.SpeedCtrl  OutDataTypeStr=uint16
  Constant6 : Constant  Value=60/TaskTimeBase.SpeedCtrl  OutDataTypeStr=uint16
  Multiport Switch : MultiPortSwitch  Inputs=4  DiagnosticForDefault=None
  Interval : Outport  VectorParamsAs1DForOutWhenUnconnected=off
  wires:
  FaultCnt/1 -> Multiport Switch/1
  Constant3/1 -> Multiport Switch/2
  Constant4/1 -> Multiport Switch/3
  Constant5/1 -> Multiport Switch/4
  Constant6/1 -> Multiport Switch/5
  Multiport Switch/1 -> Interval/1

== system AppMain/PwmInTargetSpeedEval/NormalState/PwmInSpeedCtrl/DutySpeedCtrl/SpeedAndOutDelayEval/MaxSpeedLimtedByVoltage ==
  Voltage : Inport  OutDataTypeStr=int16
  1-D Lookup Table : Lookup_n-D  NumberOfTableDimensions=1  BreakpointsForDimension1=int16([170 240 320])  Table=int16([256 256 256])  TableDataTypeStr=Inherit: Inherit from 'Table data'  ExtrapMethod=Clip  InternalRulePriority=Speed  RndMeth=Simplest  InputSameDT=on
  Constant : Constant  Value=CtrlConst.SpeedCtrl.PwmIn.TargetSpeed.Full  OutDataTypeStr=int16
  Constant1 : Constant  Value=256  OutDataTypeStr=int16
  Divide : Product  Inputs=**/
  MaxSpeed : Outport  VectorParamsAs1DForOutWhenUnconnected=off
  wires:
  Voltage/1 -> 1-D Lookup Table/1
  Constant/1 -> Divide/1
  1-D Lookup Table/1 -> Divide/2
  Divide/1 -> MaxSpeed/1
  Constant1/1 -> Divide/3

== system AppMain/PwmInTargetSpeedEval/NormalState/PwmInSpeedCtrl/DutySpeedCtrl/SpeedAndOutDelayEval/SpeedCurve ==
  MaxSpeed : Inport  OutDataTypeStr=int16
  Duty : Inport  Port=2  OutDataTypeStr=uint16
  SectorIn : Inport  Port=3  OutDataTypeStr=uint16
  Duty1 : InportShadow  Port=2  OutDataTypeStr=uint16
  Relational Operator : RelationalOperator  Operator=~=  OutDataTypeStr=boolean  RndMeth=Simplest
  SectorIn1 : InportShadow  Port=3  OutDataTypeStr=uint16
  Subsystem : Subsystem
  Subsystem1 : Subsystem
  Speed : Outport  OutDataTypeStr=int16
  DelayTime : Outport  Port=2  OutDataTypeStr=uint16
  Rst : Outport  Port=3  OutDataTypeStr=boolean
  SectorOut : Outport  Port=4  OutDataTypeStr=uint16
  wires:
  SectorIn1/1 -> Relational Operator/1  "SectorIn"
  Relational Operator/1 -> Rst/1
  Subsystem/1(SectorOut) -> [SectorOut]  "SectorOut"
  SectorIn/1 -> Subsystem/1(SectorIn)  "SectorIn"
  [SectorOut] -> Relational Operator/2, SectorOut/1
  [SectorOut] -> Subsystem1/1(SectorIn)
  MaxSpeed/1 -> Subsystem1/2(MaxSpeed)
  Duty/1 -> Subsystem1/3(Duty)  "Duty"
  Subsystem1/1(Speed) -> Speed/1
  Subsystem1/2(DelayTime) -> DelayTime/1
  Duty1/1 -> Subsystem/2(Duty)  "Duty"

== system AppMain/PwmInTargetSpeedEval/NormalState/PwmInSpeedCtrl/PwmInNotShort/DutyFilter/Enabled Subsystem ==
  Duty : Inport
  DutyLast : Inport  Port=2  OutDataTypeStr=uint16
  DutyBufIn : Inport  Port=3
  Enable : EnablePort
  DutyFilter : Subsystem
      settings: RTWFcnNameOpts=Use subsystem name
  FilteredDuty : Outport  VectorParamsAs1DForOutWhenUnconnected=off
  Valid : Outport  Port=2  VectorParamsAs1DForOutWhenUnconnected=off
  DutyBufOut : Outport  Port=3  VectorParamsAs1DForOutWhenUnconnected=off
  wires:
  DutyFilter/3(Valid) -> Valid/1
  DutyFilter/1(FilteredDuty) -> FilteredDuty/1  "FilteredDuty"
  DutyLast/1 -> DutyFilter/2(FilteredDutyLast)  "DutyLast"
  Duty/1 -> DutyFilter/1(Duty)  "Duty"
  DutyBufIn/1 -> DutyFilter/3(DutyBufIn)  "Duty"
  DutyFilter/2(DutyBufOut) -> DutyBufOut/1

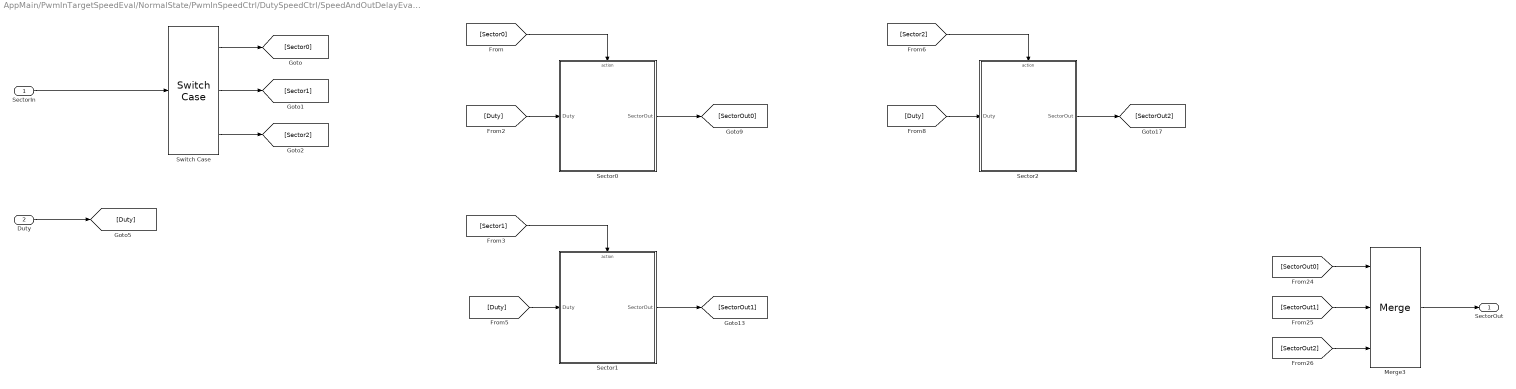
== system AppMain/PwmInTargetSpeedEval/NormalState/PwmInSpeedCtrl/DutySpeedCtrl/SpeedAndOutDelayEval/SpeedCurve/Subsystem ==
  SectorIn : Inport
  Duty : Inport  Port=2  OutDataTypeStr=uint16
  Merge3 : Merge  Inputs=3
  Sector0 : Subsystem  TreatAsAtomicUnit=on
  Sector1 : Subsystem  TreatAsAtomicUnit=on
  Sector2 : Subsystem  TreatAsAtomicUnit=on
  Switch Case : SwitchCase  CaseConditions={0,1}
  SectorOut : Outport
  wires:
  [Sector1] -> Sector1/Action
  [SectorOut0] -> Merge3/1
  Sector1/1(SectorOut) -> [SectorOut1]
  [Duty] -> Sector1/1(Duty)
  SectorIn/1 -> Switch Case/1
  [SectorOut2] -> Merge3/3
  [SectorOut1] -> Merge3/2
  Sector2/1(SectorOut) -> [SectorOut2]
  Sector0/1(SectorOut) -> [SectorOut0]
  Switch Case/3 -> [Sector2]
  [Sector0] -> Sector0/Action
  Switch Case/2 -> [Sector1]
  [Sector2] -> Sector2/Action
  [Duty] -> Sector0/1(Duty)
  [Duty] -> Sector2/1(Duty)
  Switch Case/1 -> [Sector0]
  Merge3/1 -> SectorOut/1
  Duty/1 -> [Duty]

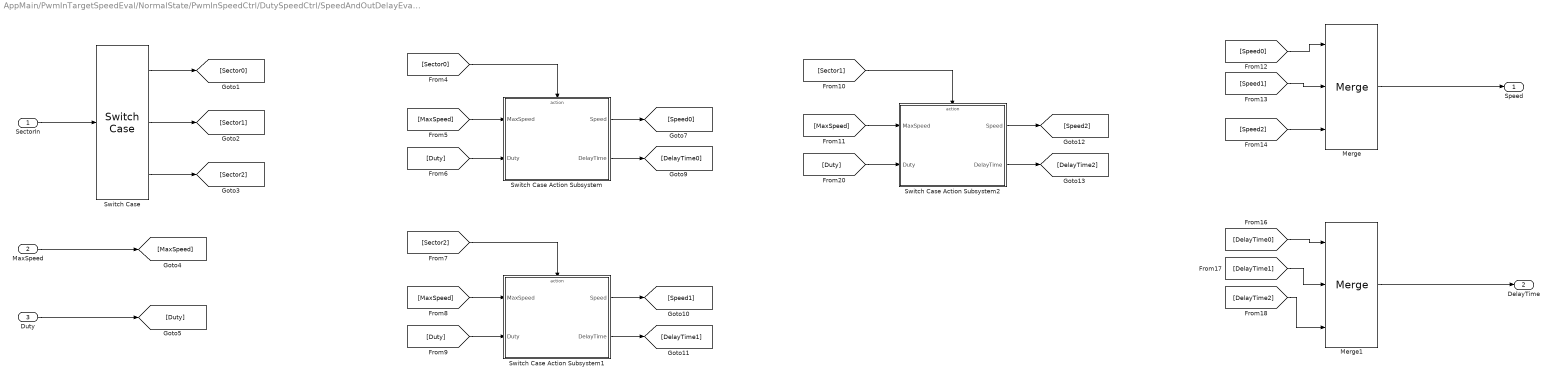
== system AppMain/PwmInTargetSpeedEval/NormalState/PwmInSpeedCtrl/DutySpeedCtrl/SpeedAndOutDelayEval/SpeedCurve/Subsystem1 ==
  SectorIn : Inport
  MaxSpeed : Inport  Port=2
  Duty : Inport  Port=3
  Merge : Merge  Inputs=3
  Merge1 : Merge  Inputs=3
  Switch Case : SwitchCase  CaseConditions={0,1}
  Switch Case Action Subsystem : Subsystem  TreatAsAtomicUnit=on
  Switch Case Action Subsystem1 : Subsystem  TreatAsAtomicUnit=on
  Switch Case Action Subsystem2 : Subsystem  TreatAsAtomicUnit=on
  Speed : Outport
  DelayTime : Outport  Port=2
  wires:
  [Sector1] -> Switch Case Action Subsystem2/Action
  [DelayTime1] -> Merge1/2
  Merge/1 -> Speed/1
  [DelayTime0] -> Merge1/1
  Switch Case Action Subsystem2/2(DelayTime) -> [DelayTime2]
  Switch Case Action Subsystem/1(Speed) -> [Speed0]
  [DelayTime2] -> Merge1/3
  [Speed1] -> Merge/2
  [MaxSpeed] -> Switch Case Action Subsystem/1(MaxSpeed)
  [MaxSpeed] -> Switch Case Action Subsystem2/1(MaxSpeed)
  Switch Case Action Subsystem1/2(DelayTime) -> [DelayTime1]
  Switch Case Action Subsystem2/1(Speed) -> [Speed2]
  Switch Case Action Subsystem1/1(Speed) -> [Speed1]
  [Duty] -> Switch Case Action Subsystem2/2(Duty)
  Switch Case/1 -> [Sector0]
  MaxSpeed/1 -> [MaxSpeed]
  [Duty] -> Switch Case Action Subsystem/2(Duty)
  [Speed2] -> Merge/3
  Merge1/1 -> DelayTime/1
  [Duty] -> Switch Case Action Subsystem1/2(Duty)
  [Sector2] -> Switch Case Action Subsystem1/Action
  [MaxSpeed] -> Switch Case Action Subsystem1/1(MaxSpeed)
  Duty/1 -> [Duty]
  SectorIn/1 -> Switch Case/1
  Switch Case/3 -> [Sector2]
  [Speed0] -> Merge/1
  Switch Case Action Subsystem/2(DelayTime) -> [DelayTime0]
  Switch Case/2 -> [Sector1]
  [Sector0] -> Switch Case Action Subsystem/Action

== system AppMain/PwmInTargetSpeedEval/NormalState/PwmInSpeedCtrl/PwmInNotShort/DutyFilter/Enabled Subsystem/DutyFilter ==
  Duty : Inport  OutDataTypeStr=uint16
  FilteredDutyLast : Inport  Port=2  OutDataTypeStr=uint16
  DutyBufIn : Inport  Port=3  OutDataTypeStr=uint16
  DutyBufUpdate : MATLAB Function  TreatAsAtomicUnit=on
      settings: RTWFcnNameOpts=Use subsystem name
  DutyInvalid : Subsystem  TreatAsAtomicUnit=on
  DutyMax : Constant  Value=1000  OutDataTypeStr=uint16
  DutyValid : Subsystem  TreatAsAtomicUnit=on
  If : If  IfExpression=u1 == 0
  Logical Operator : Logic  Inputs=1  AllPortsSameDT=off  OutDataTypeStr=boolean
  Merge1 : Merge
  Relational Operator1 : RelationalOperator  Operator=<=  OutDataTypeStr=boolean  RndMeth=Simplest
  Scope : Scope
  FilteredDuty : Outport  OutDataTypeStr=uint16  VectorParamsAs1DForOutWhenUnconnected=off
  DutyBufOut : Outport  Port=2  VectorParamsAs1DForOutWhenUnconnected=off
  Valid : Outport  Port=3  OutDataTypeStr=boolean  VectorParamsAs1DForOutWhenUnconnected=off
  wires:
  DutyBufUpdate/1(buf) -> DutyBufOut/1, DutyValid/1(DutyBuf), Relational Operator1/1
  Duty/1 -> DutyBufUpdate/2(data)  "Duty"
  DutyBufIn/1 -> DutyBufUpdate/1("buf ")
  DutyMax/1 -> Relational Operator1/2  "DutyMax"
  Relational Operator1/1 -> Logical Operator/1
  Logical Operator/1 -> If/1, Valid/1, Scope/1  "DutyValid"
  If/2 -> DutyValid/Action
  FilteredDutyLast/1 -> DutyInvalid/1(DutyLast), DutyValid/2(DutyLast)
  DutyValid/1(FilteredDuty) -> Merge1/2
  Merge1/1 -> FilteredDuty/1
  DutyInvalid/1(FilteredDuty) -> Merge1/1
  If/1 -> DutyInvalid/Action

== system AppMain/PwmInTargetSpeedEval/NormalState/PwmInSpeedCtrl/DutySpeedCtrl/SpeedAndOutDelayEval/SpeedCurve/Subsystem/Sector0 ==
  Duty : Inport  OutDataTypeStr=uint16
  Action Port : ActionPort  ActionPortLabel=case [ 0 ]:
  Compare To Constant : simulink/Logic and Bit Operations/Compare To Constant  relop=>  const=950  OutDataTypeStr=boolean
  Compare To Constant1 : simulink/Logic and Bit Operations/Compare To Constant  relop=>=  const=100  OutDataTypeStr=boolean
  Constant : Constant  Value=0  OutDataTypeStr=uint16
  Constant1 : Constant  Value=0  OutDataTypeStr=uint16
  Constant2 : Constant  OutDataTypeStr=uint16
  Switch : Switch  Criteria=u2 > Threshold
  Switch1 : Switch  Criteria=u2 > Threshold
  SectorOut : Outport  OutDataTypeStr=uint16
  wires:
  Duty/1 -> Compare To Constant1/1, Compare To Constant/1
  Compare To Constant/1 -> Switch/2
  Constant/1 -> Switch/1
  Switch1/1 -> Switch/3
  Constant1/1 -> Switch1/3
  Compare To Constant1/1 -> Switch1/2
  Constant2/1 -> Switch1/1
  Switch/1 -> SectorOut/1

== system AppMain/PwmInTargetSpeedEval/NormalState/PwmInSpeedCtrl/DutySpeedCtrl/SpeedAndOutDelayEval/SpeedCurve/Subsystem/Sector1 ==
  Duty : Inport  OutDataTypeStr=uint16
  Action Port : ActionPort  ActionPortLabel=case [ 1 ]:
  Compare To Constant : simulink/Logic and Bit Operations/Compare To Constant  relop=>  const=950  OutDataTypeStr=boolean
  Compare To Constant1 : simulink/Logic and Bit Operations/Compare To Constant  relop=<  const=100  OutDataTypeStr=boolean
  Constant : Constant  OutDataTypeStr=uint16
  Constant1 : Constant  Value=0  OutDataTypeStr=uint16
  Switch : Switch  Criteria=u2 > Threshold
  Switch1 : Switch  Criteria=u2 > Threshold
  SectorOut : Outport  OutDataTypeStr=uint16
  wires:
  Duty/1 -> Compare To Constant1/1, Compare To Constant/1
  Switch/1 -> SectorOut/1
  Compare To Constant/1 -> Switch/2
  Switch1/1 -> Switch/3
  Compare To Constant1/1 -> Switch1/2
  Constant/1 -> Switch1/3
  Constant1/1 -> Switch/1, Switch1/1

== system AppMain/PwmInTargetSpeedEval/NormalState/PwmInSpeedCtrl/DutySpeedCtrl/SpeedAndOutDelayEval/SpeedCurve/Subsystem/Sector2 ==
  Duty : Inport  OutDataTypeStr=uint16
  Action Port : ActionPort  ActionPortLabel=default:
  Constant : Constant  Value=0  OutDataTypeStr=uint16
  Terminator : Terminator
  SectorOut : Outport  OutDataTypeStr=uint16
  wires:
  Constant/1 -> SectorOut/1
  Duty/1 -> Terminator/1

== system AppMain/PwmInTargetSpeedEval/NormalState/PwmInSpeedCtrl/DutySpeedCtrl/SpeedAndOutDelayEval/SpeedCurve/Subsystem1/Switch Case Action Subsystem ==
  MaxSpeed : Inport  OutDataTypeStr=int16
  Duty : Inport  Port=2  OutDataTypeStr=uint16
  Action Port : ActionPort  ActionPortLabel=case [ 0 ]:
  Constant1 : Constant  Value=0  OutDataTypeStr=uint16
  Constant2 : Constant  Value=0  OutDataTypeStr=int16
  Terminator : Terminator
  Terminator1 : Terminator
  Speed : Outport  OutDataTypeStr=int16
  DelayTime : Outport  Port=2  OutDataTypeStr=uint16
  wires:
  Constant1/1 -> DelayTime/1
  Duty/1 -> Terminator/1
  Constant2/1 -> Speed/1
  MaxSpeed/1 -> Terminator1/1

== system AppMain/PwmInTargetSpeedEval/NormalState/PwmInSpeedCtrl/DutySpeedCtrl/SpeedAndOutDelayEval/SpeedCurve/Subsystem1/Switch Case Action Subsystem1 ==
  MaxSpeed : Inport  OutDataTypeStr=int16
  Duty : Inport  Port=2  OutDataTypeStr=uint16
  Action Port : ActionPort  ActionPortLabel=default:
  Constant : Constant  Value=0  OutDataTypeStr=int16
  Constant1 : Constant  Value=0  OutDataTypeStr=uint16
  Terminator : Terminator
  Terminator1 : Terminator
  Speed : Outport  OutDataTypeStr=int16
  DelayTime : Outport  Port=2  OutDataTypeStr=uint16
  wires:
  Duty/1 -> Terminator/1
  Constant1/1 -> DelayTime/1
  Constant/1 -> Speed/1
  MaxSpeed/1 -> Terminator1/1

== system AppMain/PwmInTargetSpeedEval/NormalState/PwmInSpeedCtrl/DutySpeedCtrl/SpeedAndOutDelayEval/SpeedCurve/Subsystem1/Switch Case Action Subsystem2 ==
  MaxSpeed : Inport  OutDataTypeStr=int16
  Duty : Inport  Port=2  OutDataTypeStr=uint16
  Action Port : ActionPort  ActionPortLabel=case [ 1 ]:
  Add : Sum  Inputs=+-
  Add1 : Sum  Inputs=+-
  Add2 : Sum  Inputs=+-
  Add3 : Sum
  Constant : Constant  Value=CtrlConst.SpeedCtrl.PwmIn.TargetSpeed.Max  OutDataTypeStr=int16
  Constant1 : Constant  Value=0  OutDataTypeStr=uint16
  Constant2 : Constant  Value=CtrlConst.SpeedCtrl.PwmIn.TargetSpeed.Min  OutDataTypeStr=int16
  Constant3 : Constant  Value=100  OutDataTypeStr=uint16
  Constant4 : Constant  Value=900  OutDataTypeStr=uint16
  Data Type Conversion : DataTypeConversion  OutDataTypeStr=int16
  Divide : Product  Inputs=*/
  Max : MinMax  Function=max  Inputs=2
  Min : MinMax  Inputs=2
  Min1 : MinMax  Inputs=2
  Product : Product
  Speed : Outport  OutDataTypeStr=int16
  DelayTime : Outport  Port=2  OutDataTypeStr=uint16
  wires:
  Constant1/1 -> DelayTime/1
  MaxSpeed/1 -> Min/1
  Min/1 -> Data Type Conversion/1
  Constant3/1 -> Add/2, Add1/2, Max/2
  Constant4/1 -> Min1/2, Add1/1
  Constant/1 -> Add2/1
  Constant2/1 -> Add3/2, Add2/2
  Add/1 -> Product/1
  Add2/1 -> Product/2
  Product/1 -> Divide/1
  Add1/1 -> Divide/2
  Divide/1 -> Add3/1
  Add3/1 -> Min/2
  Data Type Conversion/1 -> Speed/1
  Duty/1 -> Min1/1
  Min1/1 -> Max/1
  Max/1 -> Add/1

== system AppMain/PwmInTargetSpeedEval/NormalState/PwmInSpeedCtrl/PwmInNotShort/DutyFilter/Enabled Subsystem/DutyFilter/DutyInvalid ==
  DutyLast : Inport  OutDataTypeStr=uint16
  Action Port : ActionPort  ActionPortLabel=if(u1 == 0)
  FilteredDuty : Outport  OutDataTypeStr=uint16  VectorParamsAs1DForOutWhenUnconnected=off
  wires:
  DutyLast/1 -> FilteredDuty/1

== system AppMain/PwmInTargetSpeedEval/NormalState/PwmInSpeedCtrl/PwmInNotShort/DutyFilter/Enabled Subsystem/DutyFilter/DutyValid ==
  DutyBuf : Inport  OutDataTypeStr=uint16
  DutyLast : Inport  Port=2  OutDataTypeStr=uint16
  Action Port : ActionPort  ActionPortLabel=else
  BufDataSameFirstCnt : MATLAB Function  TreatAsAtomicUnit=on
      settings: RTWFcnNameOpts=Use subsystem name
  DutySameCntTHR : Constant  Value=CtrlConst.SpeedCtrl.PwmIn.Duty.Filter.DutySameCntTHR  OutDataTypeStr=uint16  SampleTime=-1
  DutyTolerance : Constant  Value=CtrlConst.SpeedCtrl.PwmIn.Duty.Filter.DutyTolerance  OutDataTypeStr=uint16  SampleTime=-1
  Relational Operator : RelationalOperator  OutDataTypeStr=boolean  RndMeth=Simplest
  Scope : Scope  NumInputPorts=3
  Selector : Selector  IndexMode=Zero-based  InputPortWidth=6  IndexOptions=Index vector (dialog)  Indices=0  OutputSizes=1
  Switch : Switch  Criteria=u2 > Threshold
  FilteredDuty : Outport  OutDataTypeStr=uint16  VectorParamsAs1DForOutWhenUnconnected=off
  wires:
  DutyLast/1 -> Switch/3
  Switch/1 -> FilteredDuty/1, Scope/2  "FilteredDuty"
  BufDataSameFirstCnt/1(samecnt) -> Relational Operator/1, Scope/1  "SameCnt"
  Selector/1 -> Switch/1, Scope/3  "Duty0"
  Relational Operator/1 -> Switch/2
  DutySameCntTHR/1 -> Relational Operator/2
  DutyBuf/1 -> BufDataSameFirstCnt/1(buf), Selector/1
  DutyTolerance/1 -> BufDataSameFirstCnt/2(tolerance)

== matlab function AppMain/AnlogVoltageToDuty/MATLAB Function ==
  data: SectorLast input uint16; SectorNew output uint16; Voltage input uint16; Duty output uint16
function [SectorNew,Duty]  = fcn(SectorLast,Voltage)

if SectorLast == 0
    if Voltage > 20
        SectorNew = uint16(1);
    else
        SectorNew =uint16(0);
    end
else
    if Voltage <= 15
        SectorNew = uint16(0);
    else
        SectorNew = uint16(1);
    end
end

if SectorNew == 0 || SectorNew == 2
    Duty = uint16(80);
else
    if Voltage <= 20
        Duty = uint16(250);
    elseif Voltage >=100
        Duty = uint16(900);
    else
         Duty = (uint16(Voltage)-uint16(20))*uint16(900-250)/uint16(100-20)+uint16(250);
    end    
end

== stateflow chart AppMain/SleepMode/SleepMode ==
  state SleepWait
    SleepWait -> (junction 16)
    (junction 16) -> (junction 18) [order 1] : [SleepWaitTime < SleepWaitTimeTHR]
        | {SleepWaitTime = SleepWaitTime + 1;}
    (junction 16) -> (junction 22) [order 2]
    (junction 22) -> (junction 21) [order 1] : [SleepValid == true]
        | {ChipSleep = true;}
    (junction 22) -> (junction 24) [order 2] : {ChipReset = true;}
  state SleepValidFilter
    en:
    GoToSleep = false;
    ChipSleep = false;
    ChipReset = false;
    exit:
    GoToSleep = true;
    (junction 9) -> (junction 11) [order 1] : [SleepValid == true]
        | {SleepValidCnt = SleepValidCnt + 1;}
    SleepValidFilter -> (junction 9) [order 1]
    (junction 9) -> (junction 11) [order 2] : {SleepValidCnt =uint16( 0);}
  (default) -> SleepValidFilter
  SleepValidFilter -> SleepWait [order 1] : [SleepValid == true && SleepValidCnt >= SleepValidCntTHR]
      | {SleepWaitTime = uint16(1);}
  data: SleepValid input boolean; SleepWaitTime local uint16; GoToSleep output boolean; SleepValidCnt local uint16 =uint16(0); ChipSleep output boolean =false; ChipReset output boolean =false; SleepValidCntTHR input uint16; SleepWaitTimeTHR input uint16

== matlab function AppMain/PwmInTargetSpeedEval/NormalState/PwmInSpeedCtrl/PwmInNotShort/DutyFilter/Enabled Subsystem/DutyFilter/DutyBufUpdate ==
  data: buf input; data input; buf output
function buf = BufDataFirst2End(buf,data)
% # eml
len = length(buf);
for i = 0 : len -2
    buf(len - i) = buf(len - i - 1);
end

buf(1) = data;
